simulink model "Project_PeregrineFalconDive_II"  (R2020b)
settings: Solver=VariableStepAuto  StartTime=0.0  StopTime=2.5  RelTol=1e-3
StartFcn:
  | learning.simulink.clearGlows(gcs);learning.simulink.resetGraderBadge(gcs);learning.simulink.closeNotificationBar(gcs);learning.simulink.Application.getInstance().clearStateflowBreakpoints()
StopFcn:
  | save_system(gcs);learning.simulink.refreshSignalWindows
model workspace (MAT data in the model file):
  courseObject.course = 'simulink'
  courseObject.chapter = 13
  courseObject.lesson = 1
  courseObject.section = 3
  courseObject.task = 1
undefined symbols (not defined in the file): A1, A2, Cd1, Cd2, g, m, rho
CloseFcn:
  | learning.simulink.cleanupOnlineTraining
settings Model: Creator=bhuva  LastModifiedBy=bhuva
settings DataIOCC: SaveTime=off

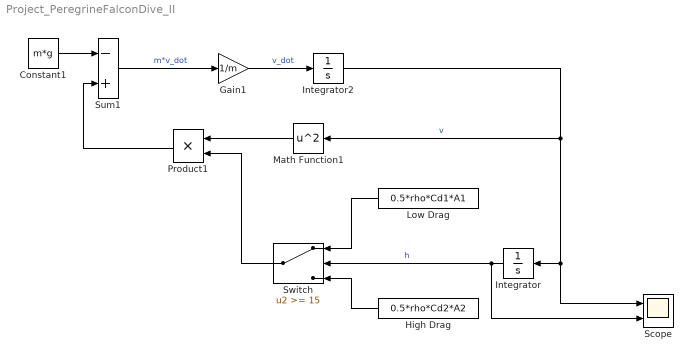
== system Project_PeregrineFalconDive_II ==
  Constant1 : Constant  Value=m*g
  Gain1 : Gain  Gain=1/m
  High Drag : Constant  Value=0.5*rho*Cd2*A2
  Integrator : Integrator  InitialCondition=60
  Integrator2 : Integrator  InitialCondition=-10
  Low Drag : Constant  Value=0.5*rho*Cd1*A1
  Math Function1 : Math  Operator=square  SignedPower=on  SaturateOnIntegerOverflow=on
  Product1 : Product
  Scope : Scope  NumInputPorts=2
  Sum1 : Sum  Inputs=-+
  Switch : Switch  Threshold=15
  wires:
  Constant1/1 -> Sum1/1
  Integrator2/1 -> Scope/1, Integrator/1, Math Function1/1  "v"
  Gain1/1 -> Integrator2/1  "v_dot"
  Product1/1 -> Sum1/2
  Sum1/1 -> Gain1/1  "m*v_dot"
  Math Function1/1 -> Product1/1
  Switch/1 -> Product1/2
  Integrator/1 -> Switch/2, Scope/2  "h"
  Low Drag/1 -> Switch/1
  High Drag/1 -> Switch/3
